simulink model "min_order"  (R2025b)
settings: Solver=VariableStepAuto  StartTime=0.0  StopTime=200  RelTol=1e-3
values from neighbouring files (symbols this model uses):
  A = [0 -0.0122335357927 0 0.04653303839 1 0 0 0 0 -2.91800139921 0 37.7525456689 ... (16 elements, 4x4)]    [matlab.mat]
  B = [0 -0.714154574773 0 -0.000498818992568]    [matlab.mat]
  C = [1 0 0 0 0 1 0 0 0 0 1 0 ... (16 elements, 4x4)]    [matlab.mat]
  K_lqr = [-1231.62178055 75.4404321566 -1810304.48785 -294623.729953]    [matlab.mat]
undefined symbols (not defined in the file or in its folder): A_obs, B_obs, C_obs, D_obs, F_obs
settings Model: Creator=shree  LastModifiedBy=shree

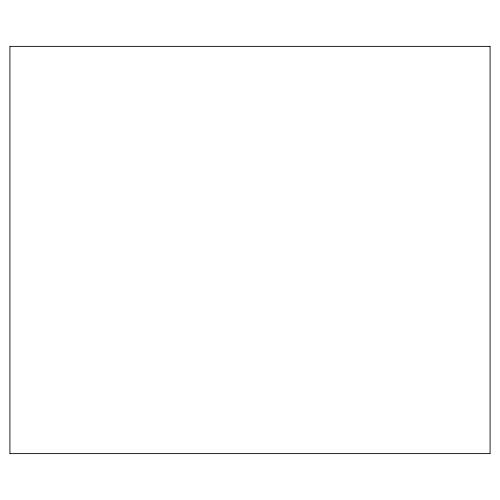
[thumbnail: Simulink's stored preview of the top-level diagram]
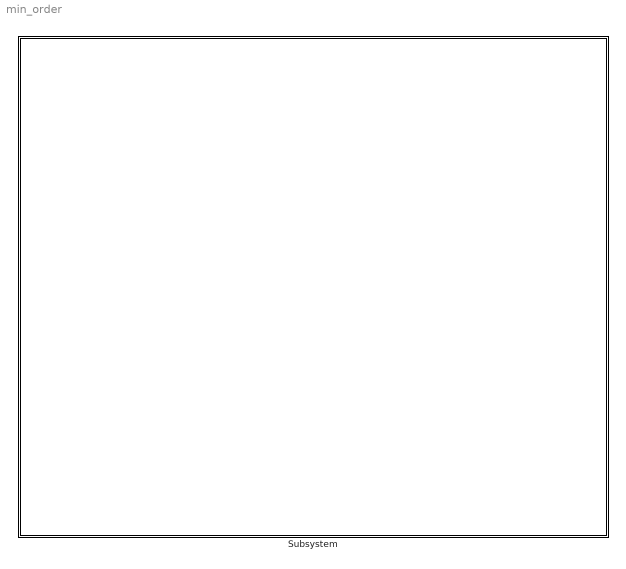
== system min_order ==
  Subsystem : Subsystem

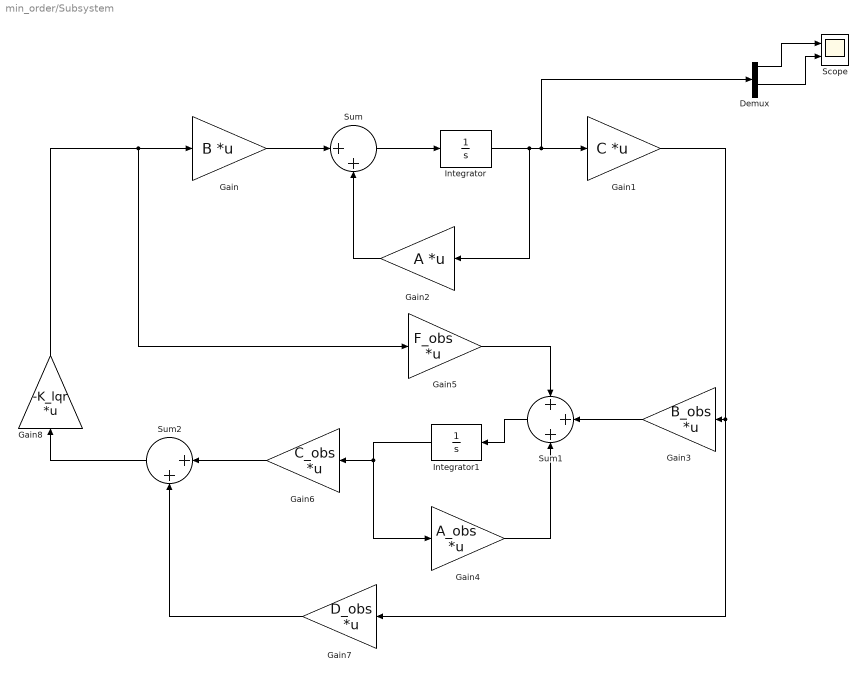
== system min_order/Subsystem ==
  Demux : Demux
  Gain : Gain  Gain=B  Multiplication=Matrix(K*u)
  Gain1 : Gain  Gain=C  Multiplication=Matrix(K*u)
  Gain2 : Gain  Gain=A  Multiplication=Matrix(K*u)
  Gain3 : Gain  Gain=B_obs  Multiplication=Matrix(K*u)
  Gain4 : Gain  Gain=A_obs  Multiplication=Matrix(K*u)
  Gain5 : Gain  Gain=F_obs  Multiplication=Matrix(K*u)
  Gain6 : Gain  Gain=C_obs  Multiplication=Matrix(K*u)
  Gain7 : Gain  Gain=D_obs  Multiplication=Matrix(K*u)
  Gain8 : Gain  Gain=-K_lqr  Multiplication=Matrix(K*u)
  Integrator : Integrator  InitialCondition=[0.01,0,0.087266,0]
  Integrator1 : Integrator  InitialCondition=[-0.02, 0 ,0]
  Scope : Scope  NumInputPorts=2
      settings: ActiveDisplayYMinimum=-0.055678573136401871  ActiveDisplayYMaximum=0.087294554178749373
  Sum : Sum  Inputs=|++
  Sum1 : Sum  Inputs=+++
  Sum2 : Sum  Inputs=|++
  wires:
  Gain/1 -> Sum/1
  Sum/1 -> Integrator/1
  Integrator/1 -> Gain2/1, Demux/1, Gain1/1
  Gain2/1 -> Sum/2
  Gain1/1 -> Gain7/1, Gain3/1
  Gain3/1 -> Sum1/2
  Gain4/1 -> Sum1/3
  Gain5/1 -> Sum1/1
  Sum1/1 -> Integrator1/1
  Integrator1/1 -> Gain4/1, Gain6/1
  Gain6/1 -> Sum2/1
  Gain7/1 -> Sum2/2
  Sum2/1 -> Gain8/1
  Gain8/1 -> Gain5/1, Gain/1
  Demux/1 -> Scope/1
  Demux/3 -> Scope/2
